simulink model "AAcontrolPIDposicion_realimentaPosicion"  (R2012b)
settings: Solver=ode45  StartTime=0.0  StopTime=5  RelTol=1e-3
values from neighbouring files (symbols this model uses):
  b_m = bm+(bl/r^2)    (= 1.5e-05)    [InicializaYconstantes.m]
  J_m = Jm+(Jl/r^2)    (= 5.65099476805e-06)    [InicializaYconstantes.m]
  Kd = J_m*n*wpos    (= 0.0113019895361)    [InicializaYconstantes.m]
  Ki = J_m*wpos^3    (= 2893.30932124)    [InicializaYconstantes.m]
  Kp = J_m*n*wpos^2    (= 9.04159162887)    [InicializaYconstantes.m]
  lambda = 0.01546    [InicializaYconstantes.m]
  Ld = 6.6*10^-3    (= 0.0066)    [InicializaYconstantes.m]
  Lq = 5.8*10^-3    (= 0.0058)    [InicializaYconstantes.m]
  Pp = 3    [InicializaYconstantes.m]
  r = 314.3008    [InicializaYconstantes.m]
  R1 = -p1i*Lq    (= 29)    [InicializaYconstantes.m]
  R2 = -p1i*Ld    (= 33)    [InicializaYconstantes.m]
  Rs = 1.02    [InicializaYconstantes.m]
  T_l = Tl/r    (= 0.00499521477515)    [InicializaYconstantes.m]
settings Model: Creator=usuario  LastModifiedBy=usuario

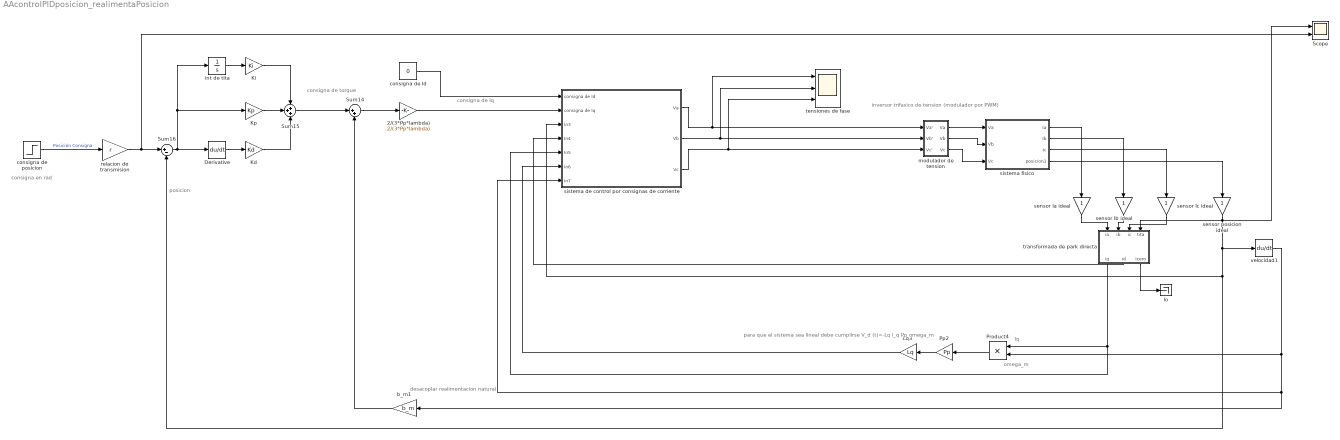
== system AAcontrolPIDposicion_realimentaPosicion ==
  note: consigna en rad
  note: posicion
  note: consigna de torque
  note: desacoplar
      | realimentacion natural
  note: consigna de Iq
  note: inversor trifasico de tension
      | (modulador por PWM)
  note: omega_m
  note: Iq
  note: para que el sistema sea lineal debe cumplirse
      | V_d (t)=-Lq  i_q  Pp omega_m
  2/(3*Pp*lambda) : Gain  Gain=2/(3*Pp*lambda)
  Derivative : Derivative
  Io : Terminator
  Kd : Gain  Gain=Kd
  Ki : Gain  Gain=Ki
  Kp : Gain  Gain=Kp
  Lq3 : Gain  Gain=Lq
  Pp2 : Gain  Gain=Pp
  Product4 : Product  RndMeth=Zero
  Scope : Scope  NumInputPorts=2
      settings: YMin=4e+06~942.902  YMax=1.7e+07~942.902  SaveName=ScopeData5
  Sum14 : Sum  Inputs=|++
  Sum15 : Sum  Inputs=+++
  Sum16 : Sum  Inputs=|+-
  b_m1 : Gain  Gain=b_m
  consigna de Id : Constant  Value=0
  consigna de posicion : Step  Time=0.1  After=2  SampleTime=0
  int de tita : Integrator
  modulador de tension : Subsystem
  relacion de transmision : Gain  Gain=r
  sensor Ia ideal : Gain
  sensor Ib ideal : Gain
  sensor Ic ideal : Gain
  sensor posicion ideal : Gain
  sistema de control por consignas de corriente : Subsystem
  sistema fisico : Subsystem
  tensiones de fase : Scope  NumInputPorts=3
      settings: TimeRange=8  YMin=-50~0~-50  YMax=50~400~50  SaveName=ScopeData3  MaxDataPoints=8000
  transformada de park directa : Subsystem
  velocidad1 : Derivative
  wires:
  sensor posicion ideal/1 -> Scope/1, velocidad1/1, sistema de control por consignas de corriente/3(In3), Sum16/2, transformada de park directa/4(tita)
  Ki/1 -> Sum15/1
  Kp/1 -> Sum15/2
  Kd/1 -> Sum15/3
  int de tita/1 -> Ki/1
  Derivative/1 -> Kd/1
  Sum16/1 -> Derivative/1, int de tita/1, Kp/1
  consigna de posicion/1 -> relacion de transmision/1  "Posición Consigna"
  sensor Ia ideal/1 -> transformada de park directa/1(ia)
  sensor Ib ideal/1 -> transformada de park directa/2(ib)
  sensor Ic ideal/1 -> transformada de park directa/3(ic)
  Product4/1 -> Pp2/1
  Pp2/1 -> Lq3/1
  modulador de tension/1(Va) -> sistema fisico/1(Va)
  modulador de tension/2(Vb) -> sistema fisico/2(Vb)
  modulador de tension/3(Vc) -> sistema fisico/3(Vc)
  sistema fisico/1(Ia) -> sensor Ia ideal/1
  sistema fisico/2(Ib) -> sensor Ib ideal/1
  sistema fisico/3(Ic) -> sensor Ic ideal/1
  sistema fisico/4(posicion1) -> sensor posicion ideal/1
  transformada de park directa/1(iq) -> sistema de control por consignas de corriente/5(In5), Product4/1
  transformada de park directa/3(Icero) -> Io/1
  sistema de control por consignas de corriente/1(Va) -> tensiones de fase/1, modulador de tension/1(Va')
  sistema de control por consignas de corriente/3(Vc) -> tensiones de fase/3, modulador de tension/3(Vc')
  sistema de control por consignas de corriente/2(Vb) -> modulador de tension/2(Vb'), tensiones de fase/2
  consigna de Id/1 -> sistema de control por consignas de corriente/1(consigna de Id)
  2/(3*Pp*lambda)/1 -> sistema de control por consignas de corriente/2(consigna de Iq)
  transformada de park directa/2(id) -> sistema de control por consignas de corriente/4(In4)
  Lq3/1 -> sistema de control por consignas de corriente/6(In6)
  velocidad1/1 -> b_m1/1, sistema de control por consignas de corriente/7(In7), Product4/2
  b_m1/1 -> Sum14/2
  Sum14/1 -> 2/(3*Pp*lambda)/1
  Sum15/1 -> Sum14/1
  relacion de transmision/1 -> Scope/2, Sum16/1

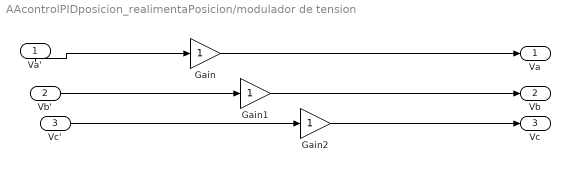
== system AAcontrolPIDposicion_realimentaPosicion/modulador de tension ==
  Va' : Inport
  Vb' : Inport  Port=2
  Vc' : Inport  Port=3
  Gain : Gain
  Gain1 : Gain
  Gain2 : Gain
  Va : Outport
  Vb : Outport  Port=2
  Vc : Outport  Port=3
  wires:
  Gain/1 -> Va/1
  Gain1/1 -> Vb/1
  Vb'/1 -> Gain1/1
  Va'/1 -> Gain/1
  Vc'/1 -> Gain2/1
  Gain2/1 -> Vc/1

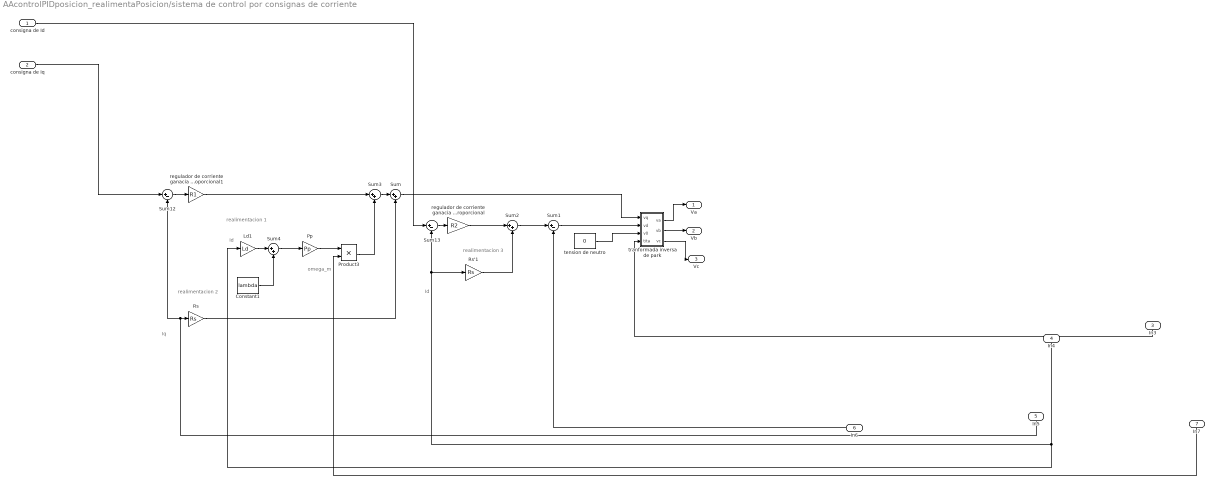
== system AAcontrolPIDposicion_realimentaPosicion/sistema de control por consignas de corriente ==
  note: Id
  note: realimentacion 3
  note: Iq
  note: realimentacion 1
  note: Id
  note: omega_m
  note: realimentacion 2
  consigna de Id : Inport
  consigna de Iq : Inport  Port=2
  In3 : Inport  Port=3
  In4 : Inport  Port=4
  In5 : Inport  Port=5
  In6 : Inport  Port=6
  In7 : Inport  Port=7
  Constant1 : Constant  Value=lambda
  Ld1 : Gain  Gain=Ld
  Pp : Gain  Gain=Pp
  Product3 : Product  RndMeth=Zero
  Rs : Gain  Gain=Rs
  Rs'1 : Gain  Gain=Rs
  Sum{,2..4} (4 alike) : Sum  Inputs=|++
  Sum1 : Sum  Inputs=|+-
  Sum12 : Sum  Inputs=|+-
  Sum13 : Sum  Inputs=|+-
  regulador de corriente ganacia proporcional : Gain  Gain=R2
  regulador de corriente ganacia proporcional1 : Gain  Gain=R1
  tension de neutro : Constant  Value=0
  tranformada inversa de park : Subsystem
  Va : Outport
  Vb : Outport  Port=2
  Vc : Outport  Port=3
  wires:
  regulador de corriente ganacia proporcional1/1 -> Sum3/1
  tension de neutro/1 -> tranformada inversa de park/3(v0)
  Sum2/1 -> Sum1/1
  Rs/1 -> Sum/2
  Sum4/1 -> Pp/1
  Constant1/1 -> Sum4/2
  Sum12/1 -> regulador de corriente ganacia proporcional1/1
  In6/1 -> Sum1/2
  Sum1/1 -> tranformada inversa de park/2(vd)
  tranformada inversa de park/1(va) -> Va/1
  tranformada inversa de park/3(vc) -> Vc/1
  Ld1/1 -> Sum4/1
  Sum/1 -> tranformada inversa de park/1(vq)
  In4/1 -> Sum13/2, Rs'1/1, Ld1/1
  Pp/1 -> Product3/1
  regulador de corriente ganacia proporcional/1 -> Sum2/1
  consigna de Id/1 -> Sum13/1
  Rs'1/1 -> Sum2/2
  consigna de Iq/1 -> Sum12/1
  tranformada inversa de park/2(vb) -> Vb/1
  Sum13/1 -> regulador de corriente ganacia proporcional/1
  Product3/1 -> Sum3/2
  Sum3/1 -> Sum/1
  In5/1 -> Sum12/2, Rs/1
  In3/1 -> tranformada inversa de park/4(tita)
  In7/1 -> Product3/2

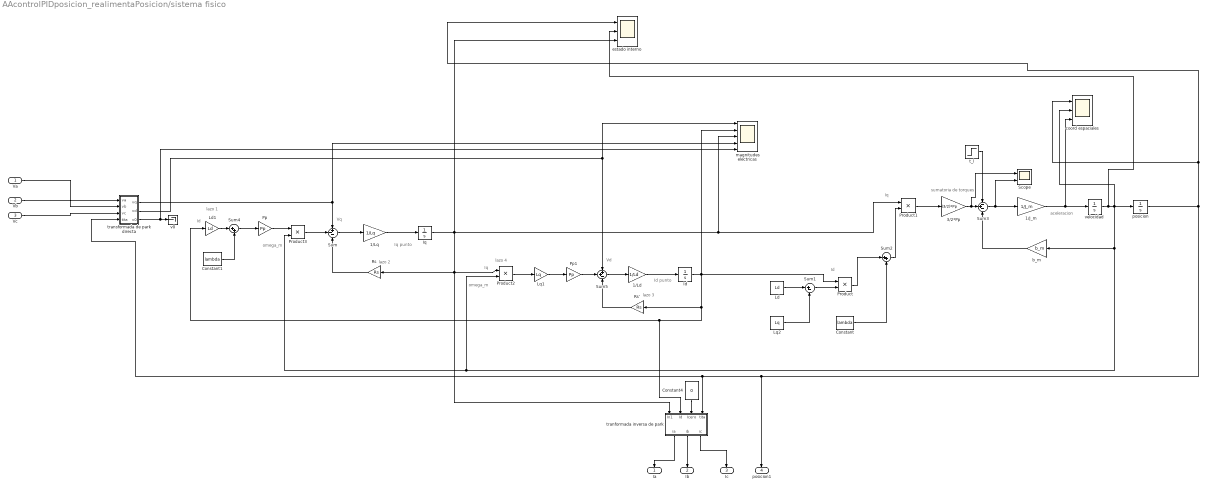
== system AAcontrolPIDposicion_realimentaPosicion/sistema fisico ==
  note: lazo 4
  note: lazo 3
  note: lazo 2
  note: lazo 1
  note: sumatoria de torques
  note: Vd
  note: omega_m
  note: Iq
  note: Id punto
  note: Vq
  note: Id
  note: Iq punto
  note: Iq
  note: aceleracion
  note: Id
  note: omega_m
  Va : Inport
  Vb : Inport  Port=2
  Vc : Inport  Port=3
  1/J_m : Gain  Gain=1/J_m
  1/Ld : Gain  Gain=1/Ld
  1/Lq : Gain  Gain=1/Lq
  3/2*Pp : Gain  Gain=(3/2)*Pp
  Constant : Constant  Value=lambda
  Constant1 : Constant  Value=lambda
  Constant4 : Constant  Value=0
  Id : Integrator
  Iq : Integrator
  Ld : Constant  Value=Ld
  Ld1 : Gain  Gain=Ld
  Lq1 : Gain  Gain=Lq
  Lq2 : Constant  Value=Lq
  Pp : Gain  Gain=Pp
  Pp1 : Gain  Gain=Pp
  Product{,1..3} (4 alike) : Product  RndMeth=Zero
  Rs : Gain  Gain=Rs
  Rs' : Gain  Gain=Rs
  Scope : Scope  NumInputPorts=2
      settings: YMin=-5~-5  YMax=5~5  SaveName=ScopeData4
  Sum : Sum  Inputs=+--
  Sum1 : Sum  Inputs=|+-
  Sum2 : Sum  Inputs=|++
  Sum3 : Sum  Inputs=-+-
  Sum4 : Sum  Inputs=|++
  Sum5 : Sum  Inputs=++-
  b_m : Gain  Gain=b_m
  coord espaciales : Scope  NumInputPorts=3
      settings: TimeRange=12  YMin=-1000~0~-50000  YMax=3000~300~100000  MaxDataPoints=8000
  estado interno : Scope  NumInputPorts=3
      settings: TimeRange=10  YMin=-2000~0~-5  YMax=6000~600~10  MaxDataPoints=8000
  magnitudes electricas : Scope  NumInputPorts=5
      settings: TimeRange=5  YMin=0~-2.5e+08~-4e+06~-1.65e+19~-1.5e+10  YMax=2.5e+17~-2.25e+08~-500000~-1.3e+19~1.5e+10  SaveName=ScopeData2  MaxDataPoints=8000
  posicion : Integrator
  t_l : Step  Time=0.3  After=T_l  SampleTime=0
  "tranformada inversa de park " : Subsystem
  transformada de park directa : Subsystem
  v0 : Terminator
  velocidad : Integrator  ContinuousStateAttributes='velocidad'
  Ia : Outport
  Ib : Outport  Port=2
  Ic : Outport  Port=3
  posicion1 : Outport  Port=4
  wires:
  Product/1 -> Sum2/1
  Ld/1 -> Sum1/1
  Lq2/1 -> Sum1/2
  Sum1/1 -> Product/2
  Constant/1 -> Sum2/2
  Sum2/1 -> Product1/2
  1/Lq/1 -> Iq/1
  Product1/1 -> 3/2*Pp/1
  Ld1/1 -> Sum4/1
  Sum3/1 -> Scope/2, 1/J_m/1
  1/Ld/1 -> Id/1
  Constant1/1 -> Sum4/2
  b_m/1 -> Sum3/3
  Sum4/1 -> Pp/1
  Sum/1 -> 1/Lq/1
  Rs/1 -> Sum/3
  t_l/1 -> Sum3/1
  Rs'/1 -> Sum5/3
  Product2/1 -> Lq1/1
  Iq/1 -> estado interno/3, magnitudes electricas/3, Product1/1, "tranformada inversa de park "/1(In1), Rs/1, Product2/1
  Lq1/1 -> Pp1/1
  Product3/1 -> Sum/2
  "tranformada inversa de park "/1(ia) -> Ia/1
  transformada de park directa/1(vq) -> magnitudes electricas/4, Sum/1
  transformada de park directa/2(vd) -> magnitudes electricas/1, Sum5/1
  "tranformada inversa de park "/2(ib) -> Ib/1
  Sum5/1 -> 1/Ld/1
  3/2*Pp/1 -> Scope/1, Sum3/2
  1/J_m/1 -> coord espaciales/3, velocidad/1
  Pp1/1 -> Sum5/2
  transformada de park directa/3(v0) -> magnitudes electricas/5, v0/1
  posicion/1 -> posicion1/1, transformada de park directa/4(tita), "tranformada inversa de park "/4(tita), estado interno/1, coord espaciales/1
  velocidad/1 -> coord espaciales/2, Product2/2, Product3/2, b_m/1, posicion/1, estado interno/2
  "tranformada inversa de park "/3(ic) -> Ic/1
  Pp/1 -> Product3/1
  Id/1 -> "tranformada inversa de park "/2(Id), Ld1/1, Rs'/1, Product/1, magnitudes electricas/2
  Constant4/1 -> "tranformada inversa de park "/3(Icero)
  Vc/1 -> transformada de park directa/3(vc)
  Vb/1 -> transformada de park directa/2(vb)
  Va/1 -> transformada de park directa/1(va)

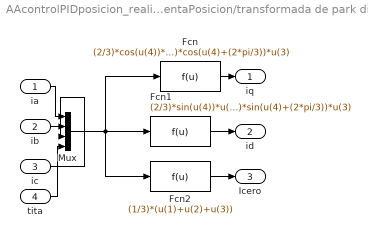
== system AAcontrolPIDposicion_realimentaPosicion/transformada de park directa ==
  ia : Inport
  ib : Inport  Port=2
  ic : Inport  Port=3
  tita : Inport  Port=4
  Fcn : Fcn  Expr=(2/3)*cos(u(4))*u(1)+(2/3)*cos(u(4)-(2*pi/3))*u(2)+(2/3)*cos(u(4)+(2*pi/3))*u(3)
  Fcn1 : Fcn  Expr=(2/3)*sin(u(4))*u(1)+(2/3)*sin(u(4)-(2*pi/3))*u(2)+(2/3)*sin(u(4)+(2*pi/3))*u(3)
  Fcn2 : Fcn  Expr=(1/3)*(u(1)+u(2)+u(3))
  Mux : Mux
  iq : Outport
  id : Outport  Port=2
  Icero : Outport  Port=3
  wires:
  Mux/1 -> Fcn1/1, Fcn/1, Fcn2/1
  Fcn/1 -> iq/1
  ia/1 -> Mux/1
  ib/1 -> Mux/2
  Fcn1/1 -> id/1
  ic/1 -> Mux/3
  tita/1 -> Mux/4
  Fcn2/1 -> Icero/1

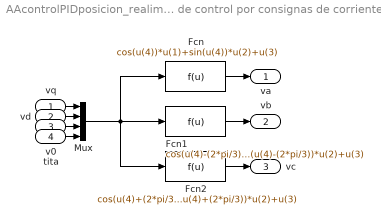
== system AAcontrolPIDposicion_realimentaPosicion/sistema de control por consignas de corriente/tranformada inversa de park ==
  vq : Inport
  vd : Inport  Port=2
  v0 : Inport  Port=3
  tita : Inport  Port=4
  Fcn : Fcn  Expr=cos(u(4))*u(1)+sin(u(4))*u(2)+u(3)
  Fcn1 : Fcn  Expr=cos(u(4)-(2*pi/3))*u(1)+sin(u(4)-(2*pi/3))*u(2)+u(3)
  Fcn2 : Fcn  Expr=cos(u(4)+(2*pi/3))*u(1)+sin(u(4)+(2*pi/3))*u(2)+u(3)
  Mux : Mux
  va : Outport
  vb : Outport  Port=2
  vc : Outport  Port=3
  wires:
  Mux/1 -> Fcn1/1, Fcn/1, Fcn2/1
  Fcn/1 -> va/1
  vq/1 -> Mux/1
  vd/1 -> Mux/2
  Fcn1/1 -> vb/1
  v0/1 -> Mux/3
  tita/1 -> Mux/4
  Fcn2/1 -> vc/1

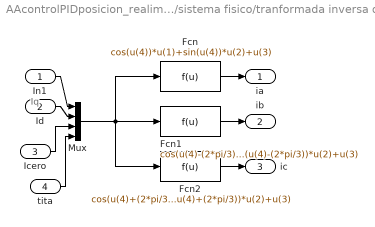
== system AAcontrolPIDposicion_realimentaPosicion/sistema fisico/tranformada inversa de park  ==
  note: Iq
  In1 : Inport
  Id : Inport  Port=2
  Icero : Inport  Port=3
  tita : Inport  Port=4
  Fcn : Fcn  Expr=cos(u(4))*u(1)+sin(u(4))*u(2)+u(3)
  Fcn1 : Fcn  Expr=cos(u(4)-(2*pi/3))*u(1)+sin(u(4)-(2*pi/3))*u(2)+u(3)
  Fcn2 : Fcn  Expr=cos(u(4)+(2*pi/3))*u(1)+sin(u(4)+(2*pi/3))*u(2)+u(3)
  Mux : Mux
  ia : Outport
  ib : Outport  Port=2
  ic : Outport  Port=3
  wires:
  Mux/1 -> Fcn1/1, Fcn/1, Fcn2/1
  Fcn/1 -> ia/1
  In1/1 -> Mux/1
  Id/1 -> Mux/2
  Fcn1/1 -> ib/1
  Icero/1 -> Mux/3
  tita/1 -> Mux/4
  Fcn2/1 -> ic/1

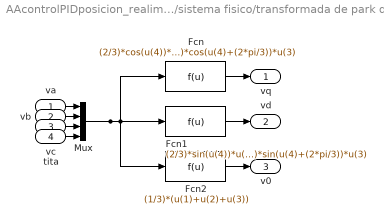
== system AAcontrolPIDposicion_realimentaPosicion/sistema fisico/transformada de park directa ==
  va : Inport
  vb : Inport  Port=2
  vc : Inport  Port=3
  tita : Inport  Port=4
  Fcn : Fcn  Expr=(2/3)*cos(u(4))*u(1)+(2/3)*cos(u(4)-(2*pi/3))*u(2)+(2/3)*cos(u(4)+(2*pi/3))*u(3)
  Fcn1 : Fcn  Expr=(2/3)*sin(u(4))*u(1)+(2/3)*sin(u(4)-(2*pi/3))*u(2)+(2/3)*sin(u(4)+(2*pi/3))*u(3)
  Fcn2 : Fcn  Expr=(1/3)*(u(1)+u(2)+u(3))
  Mux : Mux
  vq : Outport
  vd : Outport  Port=2
  v0 : Outport  Port=3
  wires:
  Mux/1 -> Fcn1/1, Fcn/1, Fcn2/1
  Fcn/1 -> vq/1
  va/1 -> Mux/1
  vb/1 -> Mux/2
  Fcn1/1 -> vd/1
  vc/1 -> Mux/3
  tita/1 -> Mux/4
  Fcn2/1 -> v0/1
